simulink model "simulinkPBLextended"  (R2020b)
settings: Solver=VariableStepAuto  StartTime=0.0  StopTime=100000  RelTol=1e-3
model workspace (MAT data in the model file):
  ON_OFF = 0
  SL_ROS_VariableLengthArrays_MaxSizes.CommonInfo.ArrayTruncateAction = 'EmitWarning'
  SL_ROS_VariableLengthArrays_MaxSizes.MsgTypeMap = containers.Map
  SL_ROS_VariableLengthArrays_MaxSizes.MsgTypeMap.serialization.keys = {'sensor_msgs/LaserScan'}
  SL_ROS_VariableLengthArrays_MaxSizes.MsgTypeMap.serialization.values{1}(1).PropertyName = 'Intensities'
  SL_ROS_VariableLengthArrays_MaxSizes.MsgTypeMap.serialization.values{1}(1).DataType = 'single'
  SL_ROS_VariableLengthArrays_MaxSizes.MsgTypeMap.serialization.values{1}(1).MaxLength = 720
  SL_ROS_VariableLengthArrays_MaxSizes.MsgTypeMap.serialization.values{1}(2).PropertyName = 'Ranges'
  SL_ROS_VariableLengthArrays_MaxSizes.MsgTypeMap.serialization.values{1}(2).DataType = 'single'
  SL_ROS_VariableLengthArrays_MaxSizes.MsgTypeMap.serialization.values{1}(2).MaxLength = 720
  SL_ROS_VariableLengthArrays_MaxSizes.MsgTypeMap.serialization.uniformity = 0
  SL_ROS_VariableLengthArrays_MaxSizes.MsgTypeMap.serialization.keyType = 'char'
  SL_ROS_VariableLengthArrays_MaxSizes.MsgTypeMap.serialization.valueType = 'any'
values from neighbouring files (symbols this model uses):
  distToReach = 0.1    [scriptPBLextended.m]
  mapSize = zeros(7,7)    [scriptPBLextended.m]
  myGoals = [  2.5   1  1;                0.2   1   0]    [scriptPBLextended.m]
  slow_ang = 0.2    [scriptPBLextended.m]
  slow_vel = 0.2    [scriptPBLextended.m]
  vizLim = [5;5;0;0]    [scriptPBLextended.m]
undefined symbols (not defined in the file or in its folder): Angular, Linear
libraries: robotlib x9, robotalgslib x2, robotcorelib x1
(part 1 of 3)
settings Model: Creator=ros  LastModifiedBy=rafal

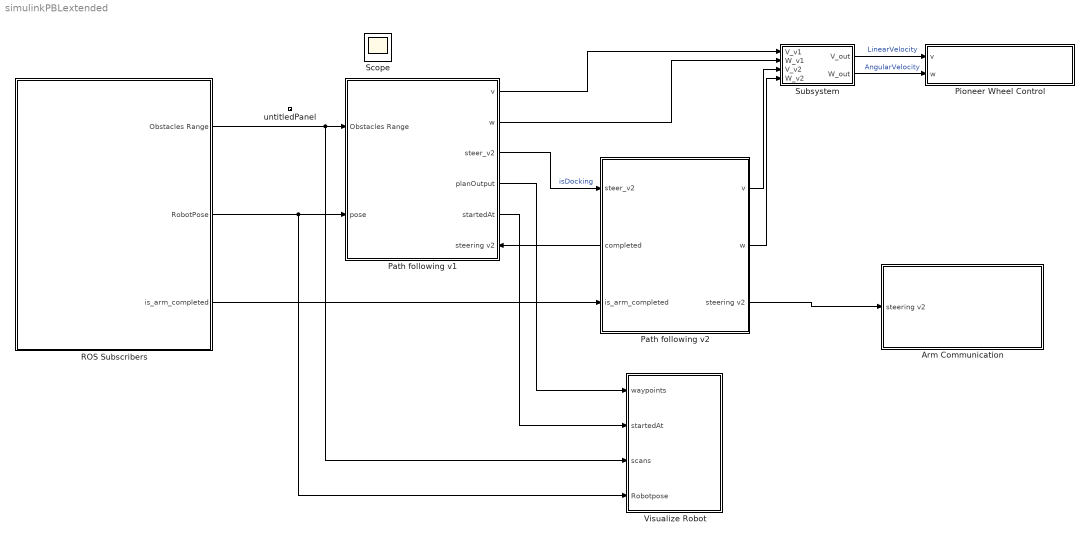
== system simulinkPBLextended ==
  Arm Communication : Subsystem
  Path following v1 : Subsystem
      settings: PortSchema="{\"entries\":[{\"content\":{\"sides\":[{\"content\":{\"connectorIds\":[\"In1\",\"In2\"]},\"type\":\"ConnectorPlacement.EquallySpacedRectSide\",\"uuid\":\"e853e1e6-c3e7-4082-99db-281a843d0b34\"},{\"content\":{\"connectorIds\":[\"Out1\",\"Out2\",\"Out3\",\"Out4\",\"Out5\",\"In3\"],\"side\":\"RIGHT\"},\"type\":\"ConnectorPlacement.EquallySpacedRectSide\",\"uuid\":\"a1f9ec42-705e-420e-9b4d-8034f0ddffe0\"},{\"content\":{\"connectorIds\":[],\"side\":\"TOP\"},\"type\":\"ConnectorPlacement.EquallySpacedRectSide\",\"uuid\":\"977e8c20-7f02-4f92-921e-d1798f70459a\"},{\"content\":{\"connectorIds\":[],\"side\":\"BOTTOM\"},\"type\":\"ConnectorPlacement.EquallySpacedRectSide\",\"uuid\":\"04f7bca2-789f-4b04-a5f5-b16c817c66c6\"},{\"content\":{\"connectorIds\":[],\"side\":\"HIDDEN\"},\"type\":\"ConnectorPlacement.EquallySpacedRectSide\",\"uuid\":\"0160847b-f5aa-4695-ad1a-b5e9ca6b09ce\"}]},\"type\":\"ConnectorPlacement.EquallySpacedConnector\",\"uuid\":\"26d10fc4-1d27-4626-95cd-b1854e221629\"}],\"packageUris\":[\"http://schema.mathworks.com/mf0/Connector/R2020b\"],\"version\":\"1.0\"}"
  Path following v2 : Subsystem
      settings: PortSchema="{\"entries\":[{\"content\":{\"sides\":[{\"content\":{\"connectorIds\":[\"In1\",\"Out4\",\"In2\"]},\"type\":\"ConnectorPlacement.EquallySpacedRectSide\",\"uuid\":\"f355e324-5119-40fb-8da4-619c1414076b\"},{\"content\":{\"connectorIds\":[\"Out1\",\"Out2\",\"Out3\"],\"side\":\"RIGHT\"},\"type\":\"ConnectorPlacement.EquallySpacedRectSide\",\"uuid\":\"4450de83-3eb5-4fdc-850c-34c402747f74\"},{\"content\":{\"connectorIds\":[],\"side\":\"TOP\"},\"type\":\"ConnectorPlacement.EquallySpacedRectSide\",\"uuid\":\"734dfc0d-eb2d-472b-b75c-9c2190a5e34b\"},{\"content\":{\"connectorIds\":[],\"side\":\"BOTTOM\"},\"type\":\"ConnectorPlacement.EquallySpacedRectSide\",\"uuid\":\"89f0bd6a-d24a-4660-95a9-6928b07425c9\"},{\"content\":{\"connectorIds\":[],\"side\":\"HIDDEN\"},\"type\":\"ConnectorPlacement.EquallySpacedRectSide\",\"uuid\":\"750f0ea6-55ba-4de2-b46c-2f888d684722\"}]},\"type\":\"ConnectorPlacement.EquallySpacedConnector\",\"uuid\":\"1650b160-7d29-44c3-8593-6b71279fd7a3\"}],\"packageUris\":[\"http://schema.mathworks.com/mf0/Connector/R2020b\"],\"version\":\"1.0\"}"
  Pioneer Wheel Control : Subsystem
  ROS Subscribers : Subsystem
  Subsystem : Subsystem
  Visualize Robot : Subsystem  mask{MeshSelectionIdx=Ground vehicle, PresetViews=Entire Map, ShowViz=on, ShowPaths=on, MapXMin=-7, MapXMax=7, MapYMin=-7, MapYMax=7, XLimits=[-size(mapSize,1) size(mapSize, 1)], YLimits=[-size(mapSize,2) size(mapSize, 2)], LocalXLimits=[-10 10], LocalYLimits=[-10 10], VisualizationSampleRate=5}
      mask prompts: MeshSelectionIdx "Robot mesh"; PresetViews "Preset Views"; ShowViz "Update visualization:"; ShowPaths "Show planned paths:"; MapXMin "Map xmin:"; MapXMax "Map xmax:"; MapYMin "Map ymin:"; MapYMax "Map ymax:"; XLimits "Map x-limits:"; YLimits "Map y-limits:"; LocalXLimits "Local view x-limits"; LocalYLimits "Local view y-limits"; VisualizationSampleRate "Sample time:"
      mask init:
      | % Create the list of key locations
      | % shelfLocationMatrix = evalin('base', get_param(gcb, 'UnloadingStation'));
      | % dockLocationMatrix = evalin('base', get_param(gcb, 'SortingStation'));
      | % 
      | % % Create popup list from matrices
      | % dockLocationNameCell = cell(size(dockLocationMatrix,1),1);
      | % shelfLocationNameCell = cell(size(shelfLocationMatrix,1),1);
      | % 
      | % for j = 1:size(shelfLocationMatrix,1)
      | %     shelfLocationNameCell{j} = ['1st Station ' num2str(j)];
      | % end
      | % for k = 1:size(dockLocationMatrix,1)
      | %     dockLocationNameCell{k} = ['2nd Station ' num2str(k)];
      | % end
      | 
      | % Update the parameter list
      | m = Simulink.Mask.get(gcb);
      | viewPopupParam = m.getParameter('PresetViews');
      | viewPopupParam.TypeOptions = [...
      |     {'Entire Map'}... %; ...
      |     %dockLocationNameCell; ...
      |     %shelfLocationNameCell 
      |     ];
      mask TypeOptions MeshSelectionIdx: Ground vehicle | Forklift
      mask TypeOptions PresetViews: Entire Map
      mask Callback PresetViews:
      | % Get key numeric data
      | % startLocationMatrix = evalin('base', get_param(gcb, 'SortingStation'));
      | % dockLocationMatrix = evalin('base', get_param(gcb, 'SortingStation'));
      | % shelfLocationMatrix = evalin('base', get_param(gcb, 'UnloadingStation'));
      | mapXLim = evalin('base', get_param(gcb, 'XLimits'));
      | mapYLim = evalin('base', get_param(gcb, 'YLimits'));
      | viewXLim = evalin('base', get_param(gcb, 'LocalXLimits'));
      | viewYLim = evalin('base', get_param(gcb, 'LocalYLimits'));
      | 
      | % Get selected value
      | viewSelection = get_param(gcb, 'PresetViews');
      | 
      | %Take action based on view
      | if strcmp(viewSelection, 'Custom')
      |     % Do nothing
      | else
      | %    if strcmp(viewSelection(1:5), 'Charg')
      |         % Start location
      |     %    startIndex = str2double(viewSelection(end));
      |    %     localPts = startLocationMatrix(startIndex, :);
      |   %      viewLimits = [localPts(1)+viewXLim(1) localPts(1)+viewXLim(2) ...
      |  %           localPts(2)+viewYLim(1) localPts(2)+viewYLim(2)];
      | %
      | %    elseif strcmp(viewSelection(1:5), 'Sorti')
      |         % Dock (Loading) location
      |     %    dockIndex = str2double(viewSelection(end));
      |    %     localPts = dockLocationMatrix(dockIndex, :);
      |   %      viewLimits = [localPts(1)+viewXLim(1) localPts(1)+viewXLim(2) ...
      |  %           localPts(2)+viewYLim(1) localPts(2)+viewYLim(2)];
      | %
      | %    elseif strcmp(viewSelection(1:5), 'Unloa')
      |         % Shelf (Unloading) location
      |      %   shelfIndex = str2double(viewSelection(end));
      |     %    localPts = shelfLocationMatrix(shelfIndex, :);
      |    %     viewLimits = [localPts(1)+viewXLim(1) localPts(1)+viewXLim(2) ...
      |   %          localPts(2)+viewYLim(1) localPts(2)+viewYLim(2)];
      |  %
      |  %   else
      |         % Show the whole map
      |         viewLimits = [mapXLim(1) mapXLim(2) mapYLim(1) mapYLim(2)];
      | %     end
      | 
      |     % Set the map parameters
      |     set_param(gcb, 'MapXMin', num2str(viewLimits(1)));
      |     set_param(gcb, 'MapXMax', num2str(viewLimits(2)));
      |     set_param(gcb, 'MapYMin', num2str(viewLimits(3)));
      |     set_param(gcb, 'MapYMax', num2str(viewLimits(4)));
      | end
      mask Callback MapXMin:
      | currentMax = str2num(get_param(gcb, 'MapXMax'));
      | newMin = str2num(get_param(gcb, 'MapXMin'));
      | if newMin > currentMax
      |     set_param(gcb, 'MapXMax', num2str(newMin+1));
      | end
      mask Callback MapXMax:
      | currentMin = str2num(get_param(gcb, 'MapXMin'));
      | newMax = str2num(get_param(gcb, 'MapXMax'));
      | if newMax < currentMin
      |     set_param(gcb, 'MapXMin', num2str(newMax-1));
      | end
      mask Callback MapYMin:
      | currentMax = str2num(get_param(gcb, 'MapYMax'));
      | newMin = str2num(get_param(gcb, 'MapYMin'));
      | if newMin > currentMax
      |     set_param(gcb, 'MapYMax', num2str(newMin+1));
      | end
      mask Callback MapYMax:
      | currentMin = str2num(get_param(gcb, 'MapYMin'));
      | newMax = str2num(get_param(gcb, 'MapYMax'));
      | if newMax < currentMin
      |     set_param(gcb, 'MapYMin', num2str(newMax-1));
      | end
      mask DialogControl DescGroupVar Prompt: Visualization example helper
      mask DialogControl DescTextVar Prompt: This subsystem plots the robots and environement and allows users to change the views.
      mask DialogControl ViewLimits Prompt: View limits
      mask DialogControl ViewConfigurationGroup Prompt: View configuration:
      mask Display: disp('Visualization Helper')
  untitledPanel : Subsystem  Tag=HiddenForWebPanel  IsWebBlockPanel=on
  Scope : Scope
  wires:
  ROS Subscribers/2(RobotPose) -> Visualize Robot/4(Robotpose), Path following v1/2(pose)
  Path following v1/4(planOutput) -> Visualize Robot/1(waypoints)
  ROS Subscribers/1(Obstacles Range) -> Visualize Robot/3(scans), Path following v1/1(Obstacles Range)
  Path following v1/5(startedAt) -> Visualize Robot/2(startedAt)
  Path following v1/3(steer_v2) -> Path following v2/1(steer_v2)  "isDocking"
  Path following v2/3(steering v2) -> Arm Communication/1(steering v2)
  ROS Subscribers/3(is_arm_completed) -> Path following v2/2(is_arm_completed)
  Path following v2/4(completed) -> Path following v1/3(steering v2)
  Path following v1/1(v) -> Subsystem/1(V_v1)
  Path following v1/2(w) -> Subsystem/2(W_v1)
  Path following v2/1(v) -> Subsystem/3(V_v2)
  Path following v2/2(w) -> Subsystem/4(W_v2)
  Subsystem/1(V_out) -> Pioneer Wheel Control/1(v)  "LinearVelocity"
  Subsystem/2(W_out) -> Pioneer Wheel Control/2(w)  "AngularVelocity"

== system simulinkPBLextended/Arm Communication ==
  steering v2 : Inport
  Blank Message : robotlib/Blank Message  messageClass=Message  entityType=std_msgs/Bool  messageType=std_msgs/Bool  SampleTime=inf  legacyBusStruct=off
  Bus Assignment : BusAssignment  AssignedSignals=Data
  Publish : robotlib/Publish  topicSource=Specify your own  topic=/arm_service  messageType=std_msgs/Bool  legacyBusStruct=off  messageQueueLength=1
  Subsystem : Subsystem
  wires:
  Blank Message/1 -> Bus Assignment/1
  Bus Assignment/1 -> Publish/1
  steering v2/1 -> Subsystem/1(steering v2)
  Subsystem/1(Out1) -> Bus Assignment/2

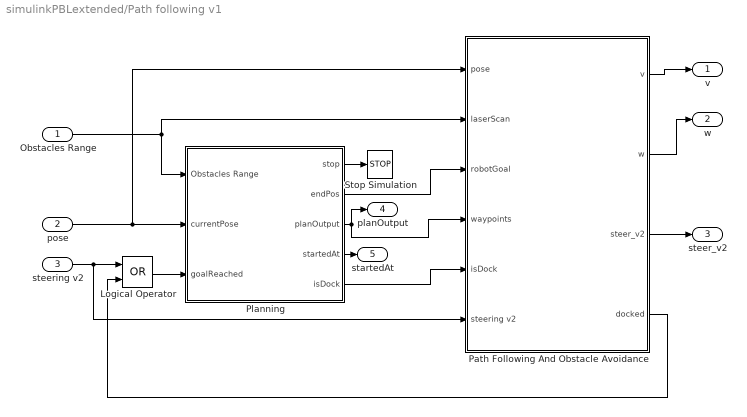
== system simulinkPBLextended/Path following v1 ==
  Obstacles Range : Inport
  pose : Inport  Port=2
  steering v2 : Inport  Port=3
  Logical Operator : Logic  Operator=OR  AllPortsSameDT=off  OutDataTypeStr=boolean
  Path Following And Obstacle Avoidance : Subsystem
  Planning : Subsystem
  Stop Simulation : Stop
  v : Outport
  w : Outport  Port=2
  steer_v2 : Outport  Port=3
  planOutput : Outport  Port=4
  startedAt : Outport  Port=5
  wires:
  Planning/4(startedAt) -> startedAt/1
  Obstacles Range/1 -> Path Following And Obstacle Avoidance/2(laserScan), Planning/1(Obstacles Range)
  Planning/1(stop) -> Stop Simulation/1
  pose/1 -> Path Following And Obstacle Avoidance/1(pose), Planning/2(currentPose)
  Path Following And Obstacle Avoidance/2(w) -> w/1
  Path Following And Obstacle Avoidance/1(v) -> v/1
  Planning/2(endPos) -> Path Following And Obstacle Avoidance/3(robotGoal)
  Logical Operator/1 -> Planning/3(goalReached)
  Planning/3(planOutput) -> Path Following And Obstacle Avoidance/4(waypoints), planOutput/1
  Planning/5(isDock) -> Path Following And Obstacle Avoidance/5(isDock)
  Path Following And Obstacle Avoidance/4(docked) -> Logical Operator/2
  steering v2/1 -> Path Following And Obstacle Avoidance/6(steering v2), Logical Operator/1
  Path Following And Obstacle Avoidance/3(steer_v2) -> steer_v2/1

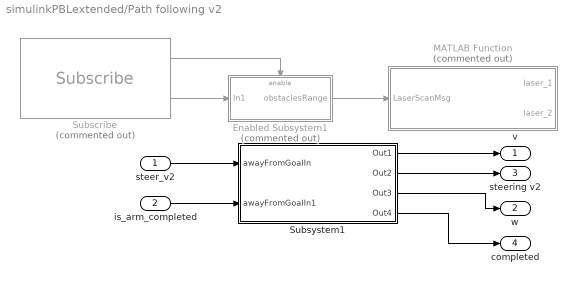
== system simulinkPBLextended/Path following v2 ==
  steer_v2 : Inport
  is_arm_completed : Inport  Port=2
  Enabled Subsystem1 : Subsystem  Commented=on  TreatAsAtomicUnit=on
  MATLAB Function : MATLAB Function  Commented=on  TreatAsAtomicUnit=on
  Subscribe : robotlib/Subscribe  Commented=on  topicSource=Specify your own  topic=/scan  messageType=sensor_msgs/LaserScan  SampleTime=-1  legacyBusStruct=off  messageQueueLength=1
  Subsystem1 : Subsystem
  v : Outport
  w : Outport  Port=2
  steering v2 : Outport  Port=3
  completed : Outport  Port=4
  wires:
  Enabled Subsystem1/1(obstaclesRange) -> MATLAB Function/1(LaserScanMsg)
  Subscribe/1 -> Enabled Subsystem1/Enable
  Subscribe/2 -> Enabled Subsystem1/1(In1)
  steer_v2/1 -> Subsystem1/1(awayFromGoalIn)
  is_arm_completed/1 -> Subsystem1/2(awayFromGoalIn1)
  Subsystem1/1(Out1) -> v/1
  Subsystem1/2(Out2) -> steering v2/1
  Subsystem1/3(Out3) -> w/1
  Subsystem1/4(Out4) -> completed/1

== system simulinkPBLextended/Pioneer Wheel Control ==
  v : Inport
  w : Inport  Port=2
  Blank Message : robotlib/Blank Message  messageClass=Message  entityType=geometry_msgs/Twist  messageType=geometry_msgs/Twist  SampleTime=inf  legacyBusStruct=off
  Bus Assignment : BusAssignment  AssignedSignals=Linear.X,Angular.Z
  Publish : robotlib/Publish  topicSource=Specify your own  topic=/diff_drive/cmd_vel  messageType=geometry_msgs/Twist  legacyBusStruct=off  messageQueueLength=1
  Subsystem : Subsystem
  Subsystem1 : Subsystem
  wires:
  Bus Assignment/1 -> Publish/1
  Blank Message/1 -> Bus Assignment/1
  v/1 -> Subsystem/1(In1)
  Subsystem/1(Out1) -> Bus Assignment/2
  w/1 -> Subsystem1/1(w)
  Subsystem1/1(Out1) -> Bus Assignment/3

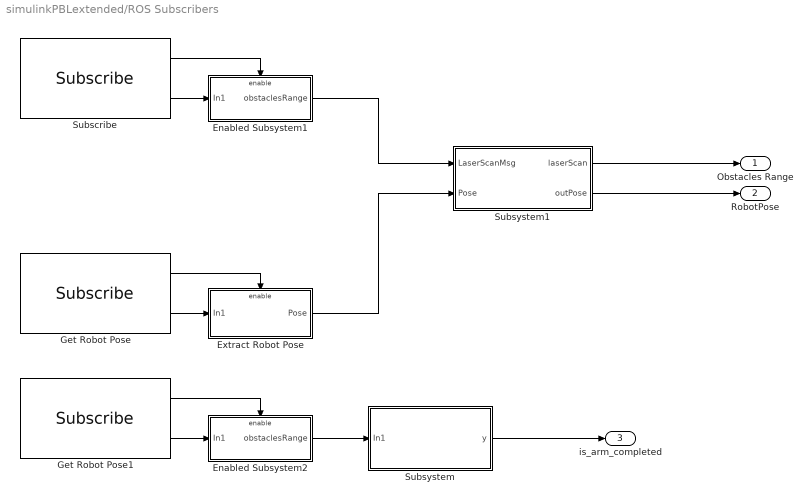
== system simulinkPBLextended/ROS Subscribers ==
  Enabled Subsystem1 : Subsystem  TreatAsAtomicUnit=on
  Enabled Subsystem2 : Subsystem  TreatAsAtomicUnit=on
  Extract Robot Pose : Subsystem
  Get Robot Pose : robotlib/Subscribe  topicSource=Specify your own  topic=/odometry/filtered  messageType=nav_msgs/Odometry  SampleTime=-1  legacyBusStruct=off  messageQueueLength=1
  Get Robot Pose1 : robotlib/Subscribe  topicSource=Specify your own  topic=/is_arm_completed  messageType=std_msgs/Bool  SampleTime=-1  legacyBusStruct=off  messageQueueLength=1
  Subscribe : robotlib/Subscribe  topicSource=Specify your own  topic=/scan  messageType=sensor_msgs/LaserScan  SampleTime=-1  legacyBusStruct=off  messageQueueLength=1
  Subsystem : Subsystem
  Subsystem1 : Subsystem
  Obstacles Range : Outport
  RobotPose : Outport  Port=2
  is_arm_completed : Outport  Port=3
  wires:
  Subscribe/2 -> Enabled Subsystem1/1(In1)
  Get Robot Pose/2 -> Extract Robot Pose/1(In1)
  Subscribe/1 -> Enabled Subsystem1/Enable
  Get Robot Pose/1 -> Extract Robot Pose/Enable
  Get Robot Pose1/1 -> Enabled Subsystem2/Enable
  Get Robot Pose1/2 -> Enabled Subsystem2/1(In1)
  Enabled Subsystem2/1(obstaclesRange) -> Subsystem/1(In1)
  Subsystem/1(y) -> is_arm_completed/1
  Enabled Subsystem1/1(obstaclesRange) -> Subsystem1/1(LaserScanMsg)
  Extract Robot Pose/1(Pose) -> Subsystem1/2(Pose)
  Subsystem1/1(laserScan) -> Obstacles Range/1
  Subsystem1/2(outPose) -> RobotPose/1

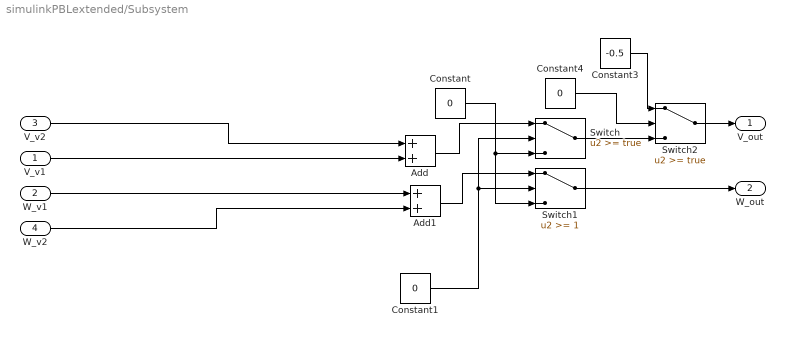
== system simulinkPBLextended/Subsystem ==
  V_v1 : Inport
  W_v1 : Inport  Port=2
  V_v2 : Inport  Port=3
  W_v2 : Inport  Port=4
  Add : Sum
  Add1 : Sum
  Constant : Constant  Value=0
  Constant1 : Constant  Value=0
  Constant3 : Constant  Value=-0.5
  Constant4 : Constant  Value=0
  Switch : Switch  Threshold=true
  Switch1 : Switch  Threshold=1
  Switch2 : Switch  Threshold=true
  V_out : Outport
  W_out : Outport  Port=2
  wires:
  W_v1/1 -> Add1/1
  V_v2/1 -> Add/1
  V_v1/1 -> Add/2
  W_v2/1 -> Add1/2
  Constant/1 -> Switch1/3, Switch/3
  Add/1 -> Switch/1
  Switch/1 -> Switch2/3
  Add1/1 -> Switch1/1
  Switch1/1 -> W_out/1
  Switch2/1 -> V_out/1
  Constant3/1 -> Switch2/1
  Constant4/1 -> Switch2/2
  Constant1/1 -> Switch1/2, Switch/2

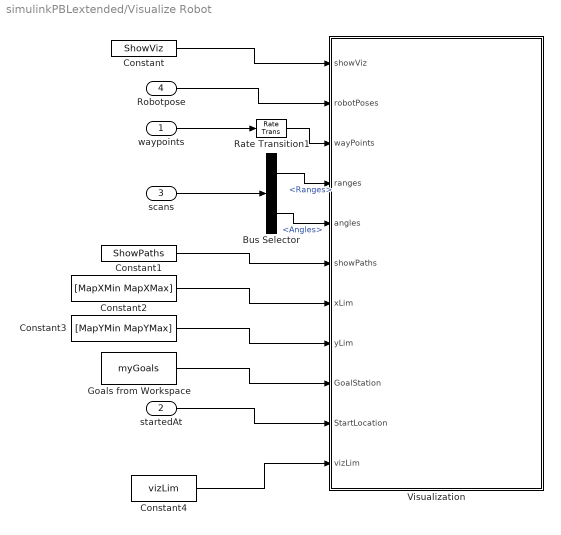
== system simulinkPBLextended/Visualize Robot ==
  waypoints : Inport
  startedAt : Inport  Port=2
  scans : Inport  Port=3
  Robotpose : Inport  Port=4
  Bus Selector : BusSelector  OutputSignals=Ranges,Angles
  Constant : Constant  Value=ShowViz
  Constant1 : Constant  Value=ShowPaths
  Constant2 : Constant  Value=[MapXMin MapXMax]
  Constant3 : Constant  Value=[MapYMin MapYMax]
  Constant4 : Constant  Value=vizLim  VectorParams1D=off
  "Goals from Workspace " : Constant  Value=myGoals  SampleTime=1
  Rate Transition1 : RateTransition
  Visualization : MATLAB Function  TreatAsAtomicUnit=on
  wires:
  Robotpose/1 -> Visualization/2(robotPoses)
  Rate Transition1/1 -> Visualization/3(wayPoints)
  Constant/1 -> Visualization/1(showViz)
  Constant1/1 -> Visualization/6(showPaths)
  Constant2/1 -> Visualization/7(xLim)
  Constant3/1 -> Visualization/8(yLim)
  waypoints/1 -> Rate Transition1/1
  scans/1 -> Bus Selector/1
  Bus Selector/1 -> Visualization/4(ranges)  "<Ranges>"
  Bus Selector/2 -> Visualization/5(angles)  "<Angles>"
  "Goals from Workspace "/1 -> Visualization/9(GoalStation)
  startedAt/1 -> Visualization/10(StartLocation)
  Constant4/1 -> Visualization/11(vizLim)
